simulink model "IBVS3Dp"  (Simulink 5.0)
settings: Solver=ode45  StartTime=0.0  StopTime=30.0  RelTol=1e-3
values from neighbouring files (symbols this model uses):
  c = camera(1000,1000,256,256,512,512)    [initHBVS.m]    (also in pose0.mat = ; pose1.mat = ; sim1.mat = ; task_endeff.mat = )
  p = reshape(u,2,n)    [CamView.m]    (also in initHBVS.m = polyhedra([0.0 0.0 0; 0.25 0.25 0; -0.25 0.25 0; -0.25 -0.25; pose0.mat = ; pose1.mat = ; sim1.mat = )
  T0c_0 = T0c    [initHBVS.m]    (also in sim1.mat = )
  T0c_x = T0c    [initHBVS.m]    (also in sim1.mat = )
  T0o =     [pose0.mat]    (also in pose1.mat; sim1.mat; task_endeff.mat; task_stereo.mat)
undefined symbols (not defined in the file or in its folder): coords, get, GetHMatrix
libraries: vs x17, simulink x3
settings Model: LastModifiedBy=ecervera  BooleanDataType=off

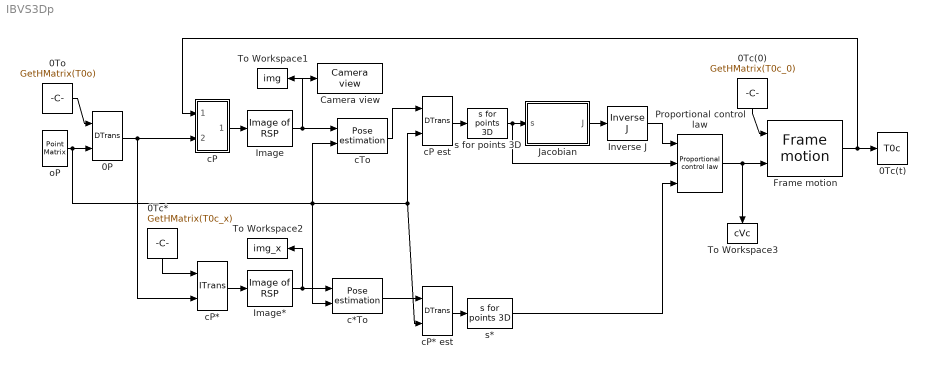
== system IBVS3Dp ==
  0P : vs/Features/DTrans  SimViewingDevice=off  DataTypeOverride=UseLocalSettings  MinMaxOverflowLogging=UseLocalSettings
      settings: Permissions=ReadWrite  RTWFcnNameOpts=Auto  RTWFileNameOpts=Auto
  0Tc(0) : Constant  Orientation=down  Value=GetHMatrix(T0c_0)  VectorParams1D=off
  0Tc(t) : ToWorkspace  VariableName=T0c  SampleTime=-1  SaveFormat=StructureWithTime
  0Tc* : Constant  Orientation=down  Value=GetHMatrix(T0c_x)  VectorParams1D=off
  0To : Constant  Value=GetHMatrix(T0o)  VectorParams1D=off
  Camera view : vs/Camera/Camera view  ms=15  em=normal  umin=0  umax=get(c,'hres')-1  vmin=0  vmax=get(c,'vres')-1  st=-1
  Frame motion : vs/Pose/Frame motion  SimViewingDevice=off  DataTypeOverride=UseLocalSettings  MinMaxOverflowLogging=UseLocalSettings
      settings: Permissions=ReadWrite  RTWFcnNameOpts=Auto  RTWFileNameOpts=Auto
  Image : vs/Camera/Image of RSP  fu=get(c,'fu')  fv=get(c,'fv')  u0=get(c,'u0')  v0=get(c,'v0')
  Image* : vs/Camera/Image of RSP  fu=get(c,'fu')  fv=get(c,'fv')  u0=get(c,'u0')  v0=get(c,'v0')
  Inverse J : vs/Jacobian/Inverse J  SimViewingDevice=off  DataTypeOverride=UseLocalSettings  MinMaxOverflowLogging=UseLocalSettings
      settings: Permissions=ReadWrite  RTWFcnNameOpts=Auto  RTWFileNameOpts=Auto
  Jacobian : Subsystem  AncestorBlock=vs/Jacobian/Jacobian of 3D points
  Proportional control law : vs/Jacobian/Proportional control law  lambda=lambda
  To Workspace1 : ToWorkspace  VariableName=img  SampleTime=-1  SaveFormat=StructureWithTime
  To Workspace2 : ToWorkspace  VariableName=img_x  SampleTime=-1  SaveFormat=StructureWithTime
  To Workspace3 : ToWorkspace  VariableName=cVc  SampleTime=-1  SaveFormat=StructureWithTime
      settings: Orientation=down
  c*To : vs/Camera/Pose estimation  fu=get(c,'fu')  fv=get(c,'fv')  u0=get(c,'u0')  v0=get(c,'v0')  threshold=0.001
  cP : Subsystem  AncestorBlock=vs/Features/ITrans
  cP est : vs/Features/DTrans  SimViewingDevice=off  DataTypeOverride=UseLocalSettings  MinMaxOverflowLogging=UseLocalSettings
      settings: Permissions=ReadWrite  RTWFcnNameOpts=Auto  RTWFileNameOpts=Auto
  cP* : vs/Features/ITrans  SimViewingDevice=off  DataTypeOverride=UseLocalSettings  MinMaxOverflowLogging=UseLocalSettings
      settings: Permissions=ReadWrite  RTWFcnNameOpts=Auto  RTWFileNameOpts=Auto
  cP* est : vs/Features/DTrans  SimViewingDevice=off  DataTypeOverride=UseLocalSettings  MinMaxOverflowLogging=UseLocalSettings
      settings: Permissions=ReadWrite  RTWFcnNameOpts=Auto  RTWFileNameOpts=Auto
  cTo : vs/Camera/Pose estimation  fu=get(c,'fu')  fv=get(c,'fv')  u0=get(c,'u0')  v0=get(c,'v0')  threshold=0.001
  oP : vs/Features/Point Matrix  m=coords(p)
  s for points 3D : vs/Jacobian/s for points 3D  SimViewingDevice=off  DataTypeOverride=UseLocalSettings  MinMaxOverflowLogging=UseLocalSettings
      settings: Permissions=ReadWrite  RTWFcnNameOpts=Auto  RTWFileNameOpts=Auto
  s* : vs/Jacobian/s for points 3D  SimViewingDevice=off  DataTypeOverride=UseLocalSettings  MinMaxOverflowLogging=UseLocalSettings
      settings: Permissions=ReadWrite  RTWFcnNameOpts=Auto  RTWFileNameOpts=Auto
  wires:
  oP/1 -> 0P/2, c*To/2, cP* est/2, cP est/2, cTo/2
  cP/1(bP) -> Image/1
  Image/1 -> Camera view/1, To Workspace1/1, cTo/1
  Jacobian/1(J) -> Inverse J/1
  Inverse J/1 -> Proportional control law/1
  s*/1 -> Proportional control law/3
  Frame motion/1 -> 0Tc(t)/1, cP/1(aTb)
  0Tc*/1 -> cP*/1
  cP*/1 -> Image*/1
  0Tc(0)/1 -> Frame motion/1
  0To/1 -> 0P/1
  0P/1 -> cP/2(aP), cP*/2
  Proportional control law/1 -> To Workspace3/1, Frame motion/2
  Image*/1 -> To Workspace2/1, c*To/1
  cTo/1 -> cP est/1
  s for points 3D/1 -> Jacobian/1(s), Proportional control law/2
  cP* est/1 -> s*/1
  c*To/1 -> cP* est/1
  cP est/1 -> s for points 3D/1

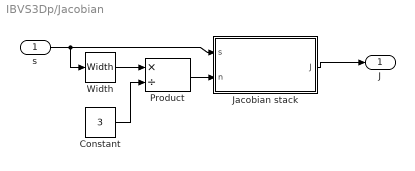
== system IBVS3Dp/Jacobian ==
  s : Inport
  Constant : Constant  Value=3
  Jacobian stack : Subsystem  TreatAsAtomicUnit=on
  Product : Product  Inputs=*/  SaturateOnIntegerOverflow=on  InputSameDT=on
  Width : Width
  J : Outport
  wires:
  Constant/1 -> Product/2
  Width/1 -> Product/1
  Product/1 -> Jacobian stack/2(n)
  s/1 -> Width/1, Jacobian stack/1(s)
  Jacobian stack/1(J) -> J/1

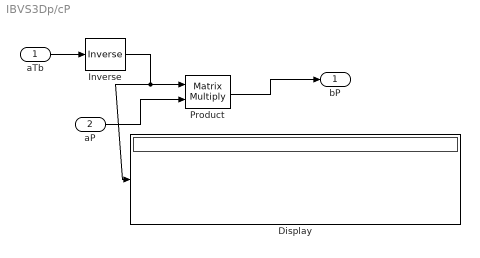
== system IBVS3Dp/cP ==
  aTb : Inport
  aP : Inport  Port=2
  Display : Display
  Inverse : vs/Pose/Inverse  SimViewingDevice=off  DataTypeOverride=UseLocalSettings  MinMaxOverflowLogging=UseLocalSettings
      settings: Permissions=ReadWrite  RTWFcnNameOpts=Auto  RTWFileNameOpts=Auto
  Product : Product  Multiplication=Matrix(*)  SaturateOnIntegerOverflow=on  InputSameDT=on
  bP : Outport
  wires:
  Inverse/1 -> Product/1, Display/1
  aTb/1 -> Inverse/1
  Product/1 -> bP/1
  aP/1 -> Product/2

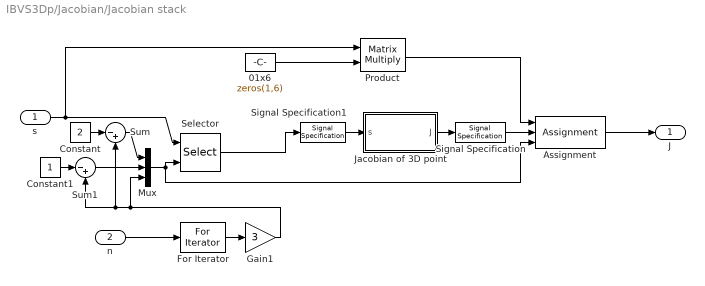
== system IBVS3Dp/Jacobian/Jacobian stack ==
  s : Inport
  n : Inport  Port=2
  01x6 : Constant  Value=zeros(1,6)  VectorParams1D=off
  Assignment : Assignment  InputType=Matrix  RowSrc=External  Columns=-1
  Constant : Constant  Value=2
  Constant1 : Constant
  For Iterator : ForIterator  IterationSource=external  OutputDataType=double
  Gain1 : Gain  Gain=3  SaturateOnIntegerOverflow=on
  Jacobian of 3D point : Subsystem
  Mux : Mux  Inputs=3
  Product : Product  Multiplication=Matrix(*)  SaturateOnIntegerOverflow=on  InputSameDT=on
  Selector : Selector  InputType=Matrix  ElementSrc=External  Elements=[1 3]  RowSrc=External  Columns=-1  InputPortWidth=3
  Signal Specification : simulink/Signal Attributes/Signal Specification  D=[3 6]  Ts=-1  DataType=auto  OutDataType=sfix(16)  OutScaling=2^0
      settings: SignalType=auto  SamplingMode=auto
  Signal Specification1 : simulink/Signal Attributes/Signal Specification  D=[3 1]  Ts=-1  DataType=auto  OutDataType=sfix(16)  OutScaling=2^0
      settings: SignalType=auto  SamplingMode=auto
  Sum : Sum  Inputs=|-+  SaturateOnIntegerOverflow=on  InputSameDT=on
  Sum1 : Sum  Inputs=|-+  SaturateOnIntegerOverflow=on  InputSameDT=on
  J : Outport
  wires:
  Sum1/1 -> Mux/2
  Constant1/1 -> Sum1/1
  s/1 -> Product/1, Selector/1
  n/1 -> For Iterator/1
  Assignment/1 -> J/1
  Product/1 -> Assignment/1
  01x6/1 -> Product/2
  Mux/1 -> Selector/2, Assignment/3
  For Iterator/1 -> Gain1/1
  Gain1/1 -> Sum1/2, Sum/2, Mux/3
  Sum/1 -> Mux/1
  Constant/1 -> Sum/1
  Jacobian of 3D point/1(J) -> Signal Specification/1
  Selector/1 -> Signal Specification1/1
  Signal Specification/1 -> Assignment/2
  Signal Specification1/1 -> Jacobian of 3D point/1(s)

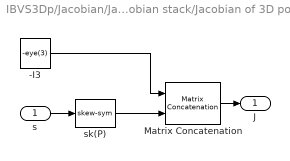
== system IBVS3Dp/Jacobian/Jacobian stack/Jacobian of 3D point ==
  s : Inport
  -I3 : Constant  Value=-eye(3)  VectorParams1D=off
  Matrix Concatenation : simulink/Math Operations/Matrix Concatenation  numInports=2  catMethod=Horizontal
  sk(P) : vs/Pose/skew-sym  SimViewingDevice=off  DataTypeOverride=UseLocalSettings  MinMaxOverflowLogging=UseLocalSettings
      settings: Permissions=ReadWrite  RTWFcnNameOpts=Auto  RTWFileNameOpts=Auto
  J : Outport
  wires:
  -I3/1 -> Matrix Concatenation/1
  sk(P)/1 -> Matrix Concatenation/2
  s/1 -> sk(P)/1
  Matrix Concatenation/1 -> J/1
